simulink model "test"  (R2013b)
settings: Solver=ode45  StartTime=0.0  StopTime=10.0  RelTol=1e-3
settings Model: Creator=z3373086  LastModifiedBy=z3373086

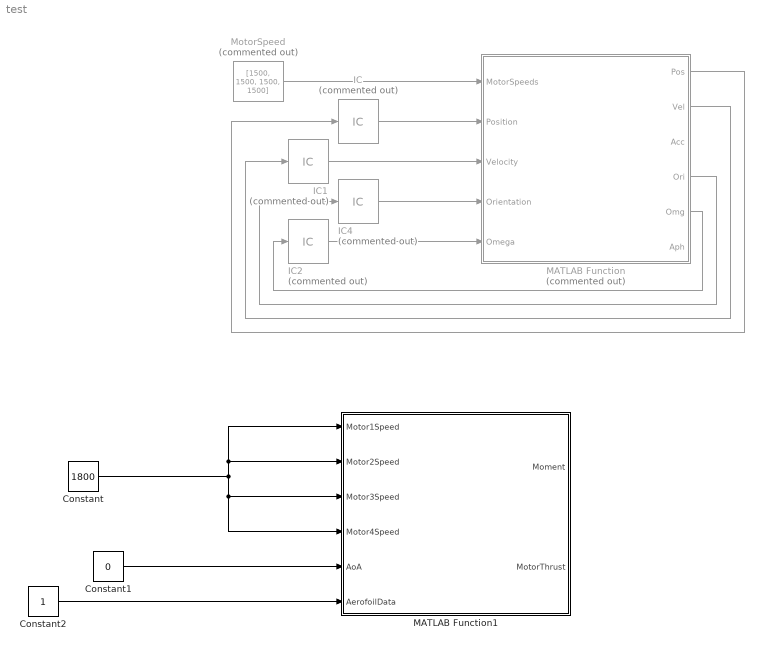
== system test ==
  Constant : Constant  Value=1800
  Constant1 : Constant  Value=0
  Constant2 : Constant
  IC{,1..2,4} (4 alike) : InitialCondition  Commented=on  Value=[0,0,0]
  MATLAB Function : MATLAB Function  Commented=on  TreatAsAtomicUnit=on
  MATLAB Function1 : MATLAB Function  TreatAsAtomicUnit=on
  MotorSpeed : Constant  Commented=on  Value=[1500, 1500, 1500, 1500]  VectorParams1D=off
  wires:
  MotorSpeed/1 -> MATLAB Function/1(MotorSpeeds)
  IC/1 -> MATLAB Function/2(Position)
  IC1/1 -> MATLAB Function/3(Velocity)
  IC4/1 -> MATLAB Function/4(Orientation)
  IC2/1 -> MATLAB Function/5(Omega)
  MATLAB Function/5(Omg) -> IC2/1
  MATLAB Function/4(Ori) -> IC4/1
  MATLAB Function/2(Vel) -> IC1/1
  MATLAB Function/1(Pos) -> IC/1
  Constant/1 -> MATLAB Function1/4(Motor4Speed), MATLAB Function1/3(Motor3Speed), MATLAB Function1/2(Motor2Speed), MATLAB Function1/1(Motor1Speed)
  Constant1/1 -> MATLAB Function1/5(AoA)
  Constant2/1 -> MATLAB Function1/6(AerofoilData)

== matlab function test/MATLAB Function1 ==
  data: Motor1Speed input; Moment output; Motor2Speed input; Motor3Speed input; Motor4Speed input; AoA input; AerofoilData input; MotorThrust output
function [Moment, MotorThrust] = SimuUpdateForces(Motor1Speed, Motor2Speed, Motor3Speed, Motor4Speed, AoA, AerofoilData)
    %Forces arising from each motor, from RPM%
    [Motor1Lift, Motor1Drag, Motor1Thrust, Motor1Torque] = MotorForces(Motor1Speed, AoA, AerofoilData);
    [Motor2Lift, Motor2Drag, Motor2Thrust, Motor2Torque] = MotorForces(Motor2Speed, AoA, AerofoilData);
    [Motor3Lift, Motor3Drag, Motor3Thrust, Motor3Torque] = MotorForces(Motor3Speed, AoA, AerofoilData);
    [Motor4Lift, Motor4Drag, Motor4Thrust, Motor4Torque] = MotorForces(Motor4Speed, AoA, AerofoilData);
    %Store these forces in vectors for each Force Type
    MotorLift = [Motor1Lift, Motor2Lift, Motor3Lift, Motor4Lift];
    MotorDrag = [Motor1Drag, Motor2Drag, Motor3Drag, Motor4Drag];
    MotorThrust = [Motor1Thrust, Motor2Thrust, Motor3Thrust, Motor4Thrust];
    MotorTorque = [Motor1Torque, Motor2Torque, Motor3Torque, Motor4Torque];
    %Calculate the Moments due to Lift Imbalances
    Moment = Moments(MotorLift, MotorTorque);
end

== matlab function test/MATLAB Function ==
  data: MotorSpeeds input; Position input; Pos output; Vel output; Velocity input; Acc output; Ori output; Omg output; Aph output; Orientation input; Omega input
function [Pos, Vel, Acc, Ori, Omg, Aph] = MainSimu(MotorSpeeds, Position, Velocity, Orientation, Omega)
%Run script to initilise varialbes and import model
AoA = 0;

%import Aerofoil Data
disp('Importing Data...');
AerofoilData = xlsread('AerofoilData');
disp('Done');

%Calculate Time increment to solve with, Initialise counters
TimeStepSize = 1/ProcessFrequency;

%Update Forces
[Moment, MotorThrust] = UpdateForces(MotorSpeeds(1), MotorSpeeds(2), MotorSpeeds(3), MotorSpeeds(4), AoA, AerofoilData);

%Update Angular Quantities
[Orientation, Omega, Alpha] = UpdateAngulars(Orientation, Omega, Moment, TimeStepSize);

%Update Translational Quantities
[Position, Velocity, Acceleration] = UpdateTranslationals(Position, Velocity, MotorThrust, Orientation, TimeStepSize);
        
Pos = Position;
Vel = Velocity;
Acc = Acceleration;
Ori = Orientation;
Omg = Omega;
Aph = Alpha;
end
